simulink model "not_sure"  (R2022b)
settings: Solver=VariableStepAuto  StartTime=0.0  StopTime=10.0  RelTol=1e-3
settings Model: Creator=Timi Banjo  LastModifiedBy=Timi Banjo

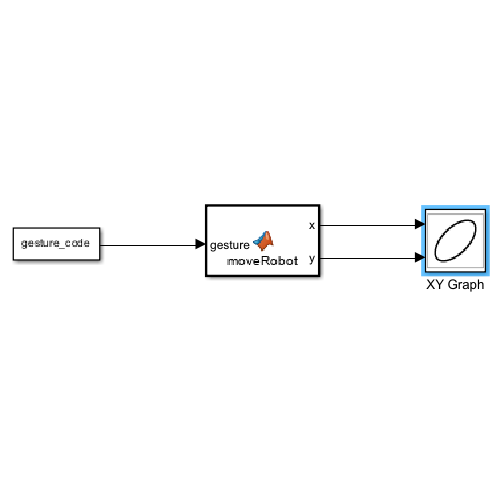
[thumbnail: Simulink's stored preview of the top-level diagram]
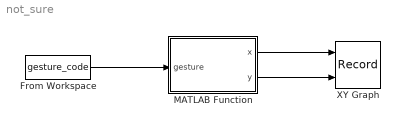
== system not_sure ==
  From Workspace : FromWorkspace  VariableName=gesture_code
  MATLAB Function : MATLAB Function  TreatAsAtomicUnit=on
  XY Graph : Record  FileSettingsInternal="{\"entries\":[{\"content\":{\"excelSettings\":{\"content\":{},\"type\":\"Streamout.ExcelSettings\"}},\"type\":\"Streamout.FileSettingStorage\",\"uuid\":\"0f0b0dc1-b5c1-4faa-8076-eea6360c50e4\"}],\"packageUris\":[\"http://schema.mathworks.com/mf0/streamout_blocks/R2020a\"],\"version\":\"1.0\"}"  Layout=[1 1]  SignalsInternal="{\"entries\":[{\"content\":{\"signals\":[{\"content\":{\"blockPath\":[\"untitled/XY Graph\"],\"channel\":[],\"dimensions\":[1],\"domain\":\"untitled/XY Graph\",\"lineColor\":\"#a2142f\",\"plots\":[1],\"port\":1,\"sid\":[\"\"],\"signalID\":427,\"signalName\":\"MATLAB Function:1\"},\"type\":\"RecordBlkView.Signal\",\"uuid\":\"1473d953-14e0-446b-b7a8-ef4117f354ee\"},{\"content\":{\"blockPath\":[\"untitled/XY Graph\"],\"channel\":[],\"dimensions\":[1],\"domain\":\"untitled/XY Graph\",\"lineColor\":\"#139fff\",\"plots\":[1],\"port\":2,\"sid\":[\"\"],\"signalID\":431,\"signalName\":\"MATLAB Function:2\"},\"type\":\"RecordBlkView.Signal\",\"uuid\":\"6059860a-02d5-44da-8624-0a47a24947c5\"}]},\"type\":\"RecordBlkView.InputSignals\",\"uuid\":\"106f1940-2a5a-450d-a981-c81e520c06c7\"}],\"packageUris\":[\"http://schema.mathworks.com/mf0/streamout_blocks/R2020a\"],\"version\":\"1.0\"}"  VisualizationBindings="{\"xyplotplugin\":{\"info\":[{\"series\":[{\"bindingParametersList\":[{\"parameter\":\"X-Axis\",\"signalID\":427,\"signalName\":\"MATLAB Function:1\"},{\"parameter\":\"Y-Axis\",\"signalID\":431,\"signalName\":\"MATLAB Function:2\"}],\"seriesID\":36605}],\"subplotID\":1}]}}"  CompatibilityTag=XY
  wires:
  From Workspace/1 -> MATLAB Function/1(gesture)
  MATLAB Function/1(x) -> XY Graph/1
  MATLAB Function/2(y) -> XY Graph/2

== matlab function not_sure/MATLAB Function ==
  data: x output; gesture input; y output
function [x, y] = moveRobot(gesture)
% Simulates robot movement based on gesture input

persistent xpos ypos angle

if isempty(xpos)
    xpos = 0;
    ypos = 0;
    angle = 0; % Facing right
end

% Motion step size
step = 0.5;

switch gesture
    case 1 % Forward
        xpos = xpos + step * cosd(angle);
        ypos = ypos + step * sind(angle);
    case 2 % Turn Left
        angle = angle + 15;
    case 3 % Turn Right
        angle = angle - 15;
    case 4 % Reverse
        xpos = xpos - step * cosd(angle);
        ypos = ypos - step * sind(angle);
    otherwise
        % Do nothing
end

x = xpos;
y = ypos;
